simulink model "simscape_quadcopter_readtime_LQR_V1_2020a"  (R2022b)
settings: Solver=ode8  StartTime=0.0  StopTime=200  FixedStep=0.002  RelTol=1e-3
values from neighbouring files (symbols this model uses):
  C = [ 1  0  0  0  0  0 ... (first row only)    [LQR_QUADCOPTER_6STATE.m]    (also in LQR_QUADCOPTER_8STATE.m = [ 1     0     0     0     0     0     0     0)
  g = 9.81    [LQR_QUADCOPTER_6STATE.m]
  K_LQR_GOC = lqr(A,B,Q,R)    [LQR_QUADCOPTER_6STATE.m]
  m = 1.7    [LQR_QUADCOPTER_6STATE.m]
  pitch_init = 0    [LQR_QUADCOPTER_6STATE.m]    (also in LQR_QUADCOPTER_8STATE.m)
  roll_init = 0    [LQR_QUADCOPTER_6STATE.m]    (also in LQR_QUADCOPTER_8STATE.m)
  v_pitch_init = 0    [LQR_QUADCOPTER_6STATE.m]    (also in LQR_QUADCOPTER_8STATE.m)
  v_roll_init = 0    [LQR_QUADCOPTER_6STATE.m]    (also in LQR_QUADCOPTER_8STATE.m)
  v_x_init = 0    [LQR_QUADCOPTER_6STATE.m]    (also in LQR_QUADCOPTER_8STATE.m)
  v_y_init = 0    [LQR_QUADCOPTER_6STATE.m]    (also in LQR_QUADCOPTER_8STATE.m)
  v_yaw_init = 0    [LQR_QUADCOPTER_6STATE.m]    (also in LQR_QUADCOPTER_8STATE.m)
  v_z_init = 0    [LQR_QUADCOPTER_6STATE.m]    (also in LQR_QUADCOPTER_8STATE.m)
  x_init = 0    [LQR_QUADCOPTER_6STATE.m]    (also in LQR_QUADCOPTER_8STATE.m)
  y_init = 0    [LQR_QUADCOPTER_6STATE.m]    (also in LQR_QUADCOPTER_8STATE.m)
  yaw_init = 0    [LQR_QUADCOPTER_6STATE.m]    (also in LQR_QUADCOPTER_8STATE.m)
  z_init = 0    [LQR_QUADCOPTER_6STATE.m]    (also in LQR_QUADCOPTER_8STATE.m)
undefined symbols (not defined in the file or in its folder): drone_leg, X, Y, Z
libraries: sm_lib x55, nesl_utility x12, simulink x1
(part 2 of 2)

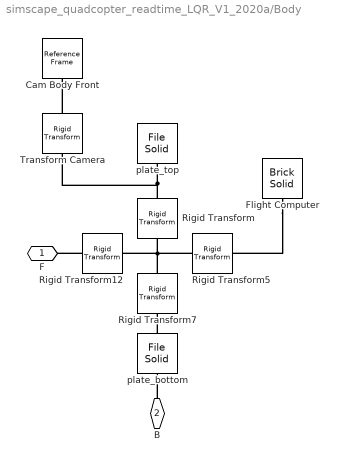
== system simscape_quadcopter_readtime_LQR_V1_2020a/Body ==
  Cam Body Front : sm_lib/Frames and Transforms/Reference Frame
  Flight Computer : sm_lib/Body Elements/Brick Solid  GraphicAmbientColor=[0.15 0.15 0.15 1.0]  BasedOnType=Mass  BrickDimensions=3*[20 20 5]  BrickDimensionUnits=mm  CenterOfMass=[0 0 0]  CenterOfMassUnits=m  GraphicDiffuseColor=[0.5 0.5 0.5]  Density=1000  DensityUnits=kg/m^3  DoExposeReferenceFrame=on  GraphicEmissiveColor=[0.0 0.0 0.0 1.0]  ExportEntireGeometry=off  SerializedFrames=<Frames/>  MarkerShape=Sphere  MarkerSize=10  GraphicType=FromGeometry  InertiaType=CalculateFromGeometry  Mass=638  MassUnits=g  MomentsOfInertia=[1 1 1]  MomentsOfInertiaUnits=kg*m^2  GraphicOpacity=1.0  ProductsOfInertia=[0 0 0]  ProductsOfInertiaUnits=kg*m^2  GraphicShininess=75  GraphicSpecularColor=[0.5 0.5 0.5 1.0]  GraphicVisPropType=SimpleVisualProperties
  Rigid Transform : sm_lib/Frames and Transforms/Rigid Transform  TranslationMethod=None  TranslationStandardOffset=0  TranslationLengthUnit=m  TranslationStandardAxis=+Z  TranslationCartesianOffset=[0 0 0]  TranslationROffset=0  TranslationROffsetUnits=m  TranslationZOffset=0  TranslationZOffsetUnits=m  TranslationThetaOffset=0  TranslationThetaOffsetUnits=deg  RotationMethod=None  RotationAngleUnits=deg  RotationStandardAxis=+Z  RotationAngle=45  RotationArbitraryAxis=[0 0 1]  FollAlignAxisA=+X  BaseAlignAxisA=+Y  FollAlignAxisB=+Y  BaseAlignAxisB=+Z  RotationSequenceAxes=FollowerAxes  RotationSequence=XYX  RotationSequenceAngles=[0 0 0]  RotationSequenceAnglesUnits=deg  RotationMatrix=[1 0 0; 0 1 0; 0 0 1]  Quaternion=[1 0 0 0]
  Rigid Transform12 : sm_lib/Frames and Transforms/Rigid Transform  TranslationMethod=Cartesian  TranslationStandardOffset=0  TranslationLengthUnit=mm  TranslationStandardAxis=+Z  TranslationCartesianOffset=[0 0 -26]  TranslationROffset=0  TranslationROffsetUnits=m  TranslationZOffset=0  TranslationZOffsetUnits=m  TranslationThetaOffset=0  TranslationThetaOffsetUnits=deg  RotationMethod=None  RotationAngleUnits=deg  RotationStandardAxis=+Z  RotationAngle=45  RotationArbitraryAxis=[0 0 1]  FollAlignAxisA=+X  BaseAlignAxisA=+Y  FollAlignAxisB=+Y  BaseAlignAxisB=+Z  RotationSequenceAxes=FollowerAxes  RotationSequence=XYX  RotationSequenceAngles=[0 0 0]  RotationSequenceAnglesUnits=deg  RotationMatrix=[1 0 0; 0 1 0; 0 0 1]  Quaternion=[1 0 0 0]
  Rigid Transform5 : sm_lib/Frames and Transforms/Rigid Transform  TranslationMethod=Cartesian  TranslationStandardOffset=0  TranslationLengthUnit=mm  TranslationStandardAxis=+Z  TranslationCartesianOffset=[0 0 -26]  TranslationROffset=0  TranslationROffsetUnits=m  TranslationZOffset=0  TranslationZOffsetUnits=m  TranslationThetaOffset=0  TranslationThetaOffsetUnits=deg  RotationMethod=None  RotationAngleUnits=deg  RotationStandardAxis=+Z  RotationAngle=45  RotationArbitraryAxis=[0 0 1]  FollAlignAxisA=+X  BaseAlignAxisA=+Y  FollAlignAxisB=+Y  BaseAlignAxisB=+Z  RotationSequenceAxes=FollowerAxes  RotationSequence=XYX  RotationSequenceAngles=[0 0 0]  RotationSequenceAnglesUnits=deg  RotationMatrix=[1 0 0; 0 1 0; 0 0 1]  Quaternion=[1 0 0 0]
  Rigid Transform7 : sm_lib/Frames and Transforms/Rigid Transform  TranslationMethod=Cartesian  TranslationStandardOffset=0  TranslationLengthUnit=mm  TranslationStandardAxis=+Z  TranslationCartesianOffset=[0 0 -38]  TranslationROffset=0  TranslationROffsetUnits=m  TranslationZOffset=0  TranslationZOffsetUnits=m  TranslationThetaOffset=0  TranslationThetaOffsetUnits=deg  RotationMethod=None  RotationAngleUnits=deg  RotationStandardAxis=+Z  RotationAngle=45  RotationArbitraryAxis=[0 0 1]  FollAlignAxisA=+X  BaseAlignAxisA=+Y  FollAlignAxisB=+Y  BaseAlignAxisB=+Z  RotationSequenceAxes=FollowerAxes  RotationSequence=XYX  RotationSequenceAngles=[0 0 0]  RotationSequenceAnglesUnits=deg  RotationMatrix=[1 0 0; 0 1 0; 0 0 1]  Quaternion=[1 0 0 0]
  Transform Camera : sm_lib/Frames and Transforms/Rigid Transform  TranslationMethod=Cartesian  TranslationStandardOffset=0  TranslationLengthUnit=m  TranslationStandardAxis=+Z  TranslationCartesianOffset=[0.06 0 0]  TranslationROffset=0  TranslationROffsetUnits=m  TranslationZOffset=0  TranslationZOffsetUnits=m  TranslationThetaOffset=0  TranslationThetaOffsetUnits=deg  RotationMethod=None  RotationAngleUnits=deg  RotationStandardAxis=+Z  RotationAngle=0.0  RotationArbitraryAxis=[0 0 1]  FollAlignAxisA=+X  BaseAlignAxisA=+Y  FollAlignAxisB=+Y  BaseAlignAxisB=+Z  RotationSequenceAxes=FollowerAxes  RotationSequence=XYX  RotationSequenceAngles=[0 0 0]  RotationSequenceAnglesUnits=deg  RotationMatrix=[1 0 0; 0 1 0; 0 0 1]  Quaternion=[1 0 0 0]
  plate_bottom : sm_lib/Body Elements/File Solid  ExtGeomFileName=C:\Users\tridu\OneDrive\Máy tính\(1)\mohinh\quadcopter_simscape\Quadcopter-Simulation-master\Quadcopter-Simulation-master\CAD\Geometry\quadcopter_drone_plate_bottom.stp  UnitType=FromFile  ExtGeomFileUnits=m  StepReaderType=HEX  ExportConvexHullGeometry=off  InertiaType=Custom  Mass=0.0317292  MassUnits=kg  CenterOfMass=[9.57262e-08, 1.0716e-07, -1.47882e-10]  CenterOfMassUnits=m  MomentsOfInertia=[2.77785e-05, 2.75764e-05, 5.53432e-05]  MomentsOfInertiaUnits=kg*m^2  ProductsOfInertia=[-9.24719e-13, -9.71809e-13, 1.0181e-10]  ProductsOfInertiaUnits=kg*m^2  BasedOnType=Density  Density=1  DensityUnits=g/cm^3  DoExposeReferenceFrame=off  SerializedFrames=<Frames><Frame><Id>Frame1</Id><Value><Name>Bot</Name><Origin><Source>GeometricFeature</Source><FeatureName>planar surface 33</FeatureName></Origin><PrimaryAxis><DefinedDirection>+Z</DefinedDirection><Source>ReferenceFrame</Source><SourceDirection>+Z</SourceDirection><FeatureName></FeatureName></PrimaryAxis><SecondaryAxis><DefinedDirection>+X</DefinedDirection><Source>ReferenceFrame</Source><SourceDirection>+Y</SourceDirection><FeatureName></FeatureName></SecondaryAxis></Value></Frame><Frame><Id>Frame2</Id><Value><Name>Top</Name><Origin><Source>ReferenceFrame</Source><FeatureName></FeatureName></Origin><PrimaryAxis><DefinedDirection>+Z</DefinedDirection><Source>ReferenceFrame</Source><SourceDirection>+Z</SourceDirection><FeatureName></FeatureName></PrimaryAxis><SecondaryAxis><DefinedDirection>+X</DefinedDirection><Source>ReferenceFrame</Source><SourceDirection>+Y</SourceDirection><FeatureName></FeatureName></SecondaryAxis></Value></Frame></Frames>  GraphicType=FromGeometry  MarkerShape=Sphere  MarkerSize=10  GraphicVisPropType=SimpleVisualProperties  GraphicDiffuseColor=[0.0 0.0 0.0]  GraphicSpecularColor=[0.5 0.5 0.5 1.0]  GraphicAmbientColor=[0.15 0.15 0.15 1.0]  GraphicEmissiveColor=[0.0 0.0 0.0 1.0]  GraphicShininess=75  GraphicOpacity=1.0
  "plate_top " : sm_lib/Body Elements/File Solid  ExtGeomFileName=C:\Users\tridu\OneDrive\Máy tính\(1)\mohinh\quadcopter_simscape\Quadcopter-Simulation-master\Quadcopter-Simulation-master\CAD\Geometry\quadcopter_drone_plate_top.stp  UnitType=FromFile  ExtGeomFileUnits=m  StepReaderType=HEX  ExportConvexHullGeometry=off  InertiaType=Custom  Mass=0.0317292  MassUnits=kg  CenterOfMass=[9.57262e-08, 1.0716e-07, -1.47882e-10]  CenterOfMassUnits=m  MomentsOfInertia=[2.77785e-05, 2.75764e-05, 5.53432e-05]  MomentsOfInertiaUnits=kg*m^2  ProductsOfInertia=[-9.24719e-13, -9.71809e-13, 1.0181e-10]  ProductsOfInertiaUnits=kg*m^2  BasedOnType=Density  Density=1  DensityUnits=g/cm^3  DoExposeReferenceFrame=on  SerializedFrames=<Frames/>  GraphicType=FromGeometry  MarkerShape=Sphere  MarkerSize=10  GraphicVisPropType=SimpleVisualProperties  GraphicDiffuseColor=[0.0 0.0 0.0]  GraphicSpecularColor=[0.5 0.5 0.5 1.0]  GraphicAmbientColor=[0.15 0.15 0.15 1.0]  GraphicEmissiveColor=[0.0 0.0 0.0 1.0]  GraphicShininess=75  GraphicOpacity=1.0
  F : PMIOPort  Side=Right
  B : PMIOPort  Port=2  Side=Left
  connections:
  Flight Computer/RConn1 -- Rigid Transform5/RConn1
  Rigid Transform7/LConn1 -- Rigid Transform5/LConn1 -- Rigid Transform12/LConn1 -- Rigid Transform/LConn1
  plate_bottom/RConn1 -- Rigid Transform7/RConn1
  Rigid Transform12/RConn1 -- F/RConn1
  Rigid Transform/RConn1 -- Transform Camera/LConn1 -- "plate_top "/RConn1
  Transform Camera/RConn1 -- Cam Body Front/RConn1
  B/RConn1 -- plate_bottom/LConn1

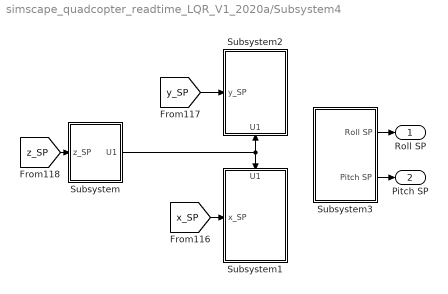
== system simscape_quadcopter_readtime_LQR_V1_2020a/Subsystem4 ==
  Subsystem : Subsystem
  Subsystem1 : Subsystem
      settings: PortSchema="{\"entries\":[{\"content\":{\"sides\":[{\"content\":{\"connectorIds\":[\"In1\"]},\"type\":\"ConnectorPlacement.EquallySpacedRectSide\",\"uuid\":\"62a51b67-9663-4f23-a0a7-17dd4d665e7c\"},{\"content\":{\"connectorIds\":[],\"side\":\"RIGHT\"},\"type\":\"ConnectorPlacement.EquallySpacedRectSide\",\"uuid\":\"9cf76029-abe2-4d70-b924-e49b8fca58fe\"},{\"content\":{\"connectorIds\":[\"In2\"],\"side\":\"TOP\"},\"type\":\"ConnectorPlacement.EquallySpacedRectSide\",\"uuid\":\"b4a1b99f-921e-474f-a2a2-454a2b8db441\"}]},\"type\":\"ConnectorPlacement.EquallySpacedConnector\",\"uuid\":\"20d905bc-00f9-441a-91aa-89485326b1f1\"}],\"packageUris\":[\"http://schema.mathworks.com/mf0/Connector/R2020b\"],\"version\":\"1.0\"}"
  Subsystem2 : Subsystem
      settings: PortSchema="{\"entries\":[{\"content\":{\"sides\":[{\"content\":{\"connectorIds\":[\"In1\"]},\"type\":\"ConnectorPlacement.EquallySpacedRectSide\",\"uuid\":\"62a51b67-9663-4f23-a0a7-17dd4d665e7c\"},{\"content\":{\"connectorIds\":[],\"side\":\"RIGHT\"},\"type\":\"ConnectorPlacement.EquallySpacedRectSide\",\"uuid\":\"9cf76029-abe2-4d70-b924-e49b8fca58fe\"},{\"content\":{\"connectorIds\":[],\"side\":\"TOP\"},\"type\":\"ConnectorPlacement.EquallySpacedRectSide\",\"uuid\":\"b4a1b99f-921e-474f-a2a2-454a2b8db441\"},{\"content\":{\"connectorIds\":[\"In2\"],\"side\":\"BOTTOM\"},\"type\":\"ConnectorPlacement.EquallySpacedRectSide\",\"uuid\":\"85e13e03-6c73-4551-a07f-9b1bfbaf7196\"}]},\"type\":\"ConnectorPlacement.EquallySpacedConnector\",\"uuid\":\"20d905bc-00f9-441a-91aa-89485326b1f1\"}],\"packageUris\":[\"http://schema.mathworks.com/mf0/Connector/R2020b\"],\"version\":\"1.0\"}"
  Subsystem3 : Subsystem
  Roll SP : Outport
  Pitch SP : Outport  Port=2
  wires:
  Subsystem3/2(Pitch SP) -> Pitch SP/1
  [z_SP] -> Subsystem/1(z_SP)
  [y_SP] -> Subsystem2/1(y_SP)
  Subsystem3/1(Roll SP) -> Roll SP/1
  [x_SP] -> Subsystem1/1(x_SP)
  Subsystem/1(U1) -> Subsystem1/2(U1), Subsystem2/2(U1)

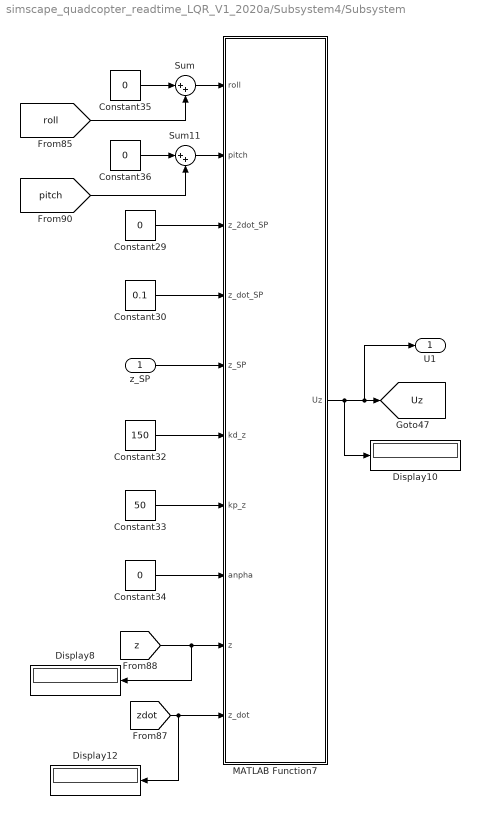
== system simscape_quadcopter_readtime_LQR_V1_2020a/Subsystem4/Subsystem ==
  z_SP : Inport
  Constant{29,34..36} (4 alike) : Constant  Value=0
  Constant30 : Constant  Value=0.1
  Constant32 : Constant  Value=150
  Constant33 : Constant  Value=50
  Display10 : Display
  Display12 : Display
  Display8 : Display
  MATLAB Function7 : MATLAB Function  TreatAsAtomicUnit=on
  Sum : Sum  Inputs=|++
  Sum11 : Sum  Inputs=|++
  U1 : Outport
  tag scope: Uz=global
  wires:
  [z] -> Display8/1, MATLAB Function7/9(z)
  Constant35/1 -> Sum/1
  Constant29/1 -> MATLAB Function7/3(z_2dot_SP)
  Constant32/1 -> MATLAB Function7/6(kd_z)
  Constant30/1 -> MATLAB Function7/4(z_dot_SP)
  [zdot] -> Display12/1, MATLAB Function7/10(z_dot)
  Sum11/1 -> MATLAB Function7/2(pitch)
  [roll] -> Sum/2
  Constant34/1 -> MATLAB Function7/8(anpha)
  Constant33/1 -> MATLAB Function7/7(kp_z)
  [pitch] -> Sum11/2
  Sum/1 -> MATLAB Function7/1(roll)
  MATLAB Function7/1(Uz) -> Display10/1, U1/1, [Uz]
  Constant36/1 -> Sum11/1
  z_SP/1 -> MATLAB Function7/5(z_SP)

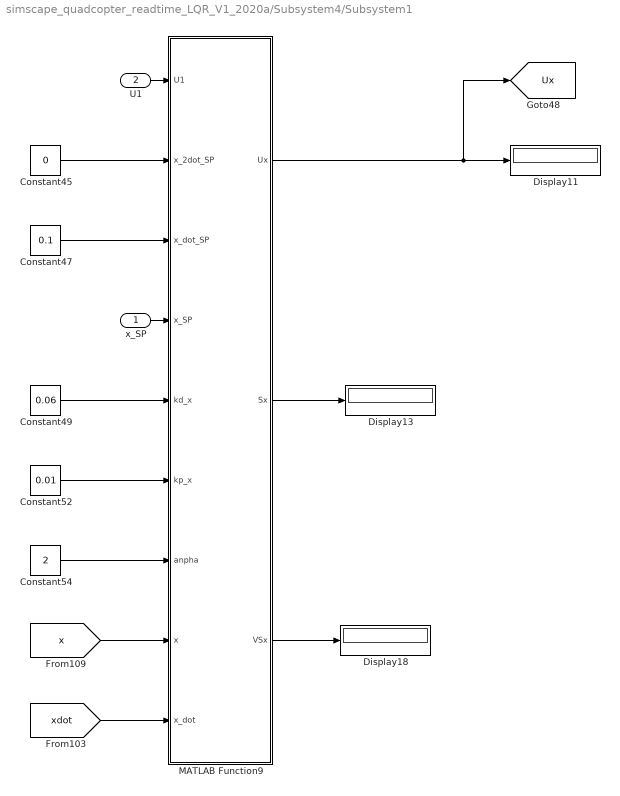
== system simscape_quadcopter_readtime_LQR_V1_2020a/Subsystem4/Subsystem1 ==
  x_SP : Inport
  U1 : Inport  Port=2
  Constant45 : Constant  Value=0
  Constant47 : Constant  Value=0.1
  Constant49 : Constant  Value=0.06
  Constant52 : Constant  Value=0.01
  Constant54 : Constant  Value=2
  Display11 : Display
  Display13 : Display
  Display18 : Display
  MATLAB Function9 : MATLAB Function  TreatAsAtomicUnit=on
  tag scope: Ux=global
  wires:
  Constant49/1 -> MATLAB Function9/5(kd_x)
  Constant54/1 -> MATLAB Function9/7(anpha)
  U1/1 -> MATLAB Function9/1(U1)
  MATLAB Function9/3(VSx) -> Display18/1
  MATLAB Function9/2(Sx) -> Display13/1
  [x] -> MATLAB Function9/8(x)
  Constant52/1 -> MATLAB Function9/6(kp_x)
  [xdot] -> MATLAB Function9/9(x_dot)
  Constant45/1 -> MATLAB Function9/2(x_2dot_SP)
  Constant47/1 -> MATLAB Function9/3(x_dot_SP)
  x_SP/1 -> MATLAB Function9/4(x_SP)
  MATLAB Function9/1(Ux) -> Display11/1, [Ux]

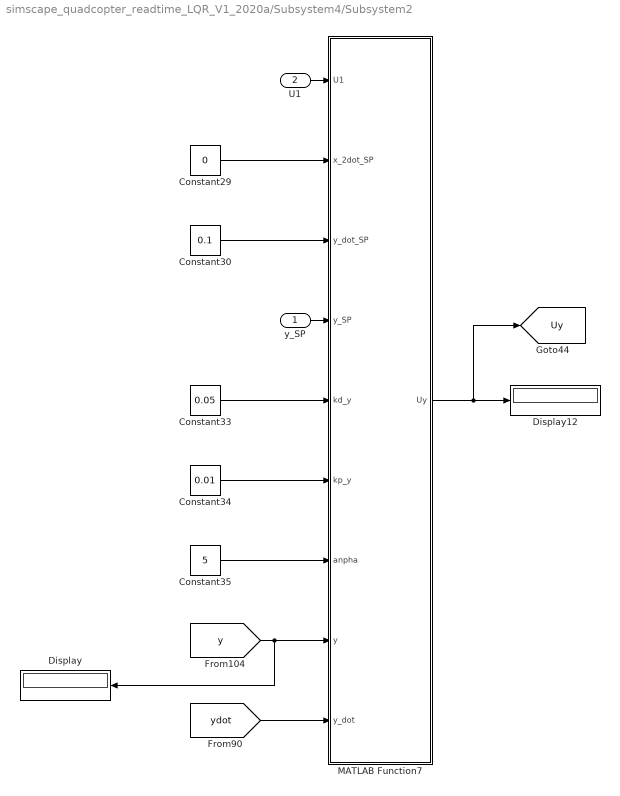
== system simscape_quadcopter_readtime_LQR_V1_2020a/Subsystem4/Subsystem2 ==
  y_SP : Inport
  U1 : Inport  Port=2
  Constant29 : Constant  Value=0
  Constant30 : Constant  Value=0.1
  Constant33 : Constant  Value=0.05
  Constant34 : Constant  Value=0.01
  Constant35 : Constant  Value=5
  Display : Display
  Display12 : Display
  MATLAB Function7 : MATLAB Function  TreatAsAtomicUnit=on
  tag scope: Uy=global
  wires:
  [ydot] -> MATLAB Function7/9(y_dot)
  Constant35/1 -> MATLAB Function7/7(anpha)
  Constant29/1 -> MATLAB Function7/2(x_2dot_SP)
  Constant34/1 -> MATLAB Function7/6(kp_y)
  MATLAB Function7/1(Uy) -> Display12/1, [Uy]
  Constant33/1 -> MATLAB Function7/5(kd_y)
  U1/1 -> MATLAB Function7/1(U1)
  Constant30/1 -> MATLAB Function7/3(y_dot_SP)
  y_SP/1 -> MATLAB Function7/4(y_SP)
  [y] -> Display/1, MATLAB Function7/8(y)

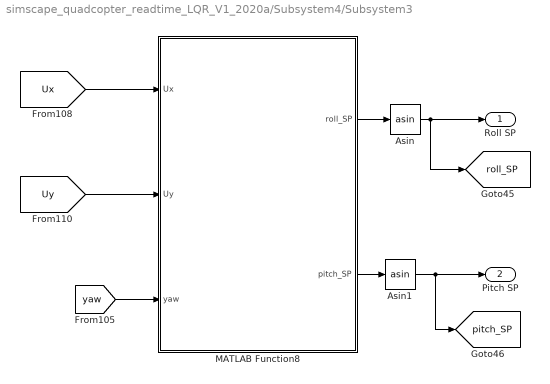
== system simscape_quadcopter_readtime_LQR_V1_2020a/Subsystem4/Subsystem3 ==
  Asin : Trigonometry  Operator=asin
  Asin1 : Trigonometry  Operator=asin
  MATLAB Function8 : MATLAB Function  TreatAsAtomicUnit=on
  Roll SP : Outport
  Pitch SP : Outport  Port=2
  tag scope: pitch_SP=global, roll_SP=global
  wires:
  [Ux] -> MATLAB Function8/1(Ux)
  [Uy] -> MATLAB Function8/2(Uy)
  MATLAB Function8/1(roll_SP) -> Asin/1
  Asin/1 -> Roll SP/1, [roll_SP]
  Asin1/1 -> [pitch_SP], Pitch SP/1
  [yaw] -> MATLAB Function8/3(yaw)
  MATLAB Function8/2(pitch_SP) -> Asin1/1

== matlab function simscape_quadcopter_readtime_LQR_V1_2020a/Subsystem4/Subsystem2/MATLAB Function7 ==
  data: U1 input; x_2dot_SP input; y_dot_SP input; y_SP input; kd_y input; kp_y input; Uy output; anpha input; y input; y_dot input
function Uy = fcn(U1,x_2dot_SP,y_dot_SP,y_SP,kd_y,kp_y,anpha,y,y_dot) 

%% khai báo biến hệ thống
m=1.7;

%% phương trình trạng thái

% y_2dot=-(U1*cos(yaw)*sin(roll) - cos(roll)*sin(pitch)*sin(yaw))/m;

%% Chọn phương trình mặt trượt có dạng

Sy=kd_y*(y_dot_SP-y_dot)+kp_y*(y_SP-y);

%% Chọn tiêu chí tốc độ hội tụ, trong đó K là hệ số dương Nếu K càng lớn thì độ hội tụ về 0 càng giảm

VSy=-anpha*abs(Sy)*sign(Sy);

%% Thiết kế tín hiệu điều khiển Ux Uy

Uy=(m/U1)*(x_2dot_SP+Sy+VSy);

end

== matlab function simscape_quadcopter_readtime_LQR_V1_2020a/Subsystem4/Subsystem1/MATLAB Function9 ==
  data: U1 input; x_2dot_SP input; x_dot_SP input; x_SP input; kd_x input; kp_x input; Ux output; anpha input; x input; x_dot input; Sx output; VSx output
function [Ux,Sx,VSx]= fcn(U1,x_2dot_SP,x_dot_SP,x_SP,kd_x,kp_x,anpha,x,x_dot) 

%% khai báo biến hệ thống

m=1.7;

%% phương trình trạng thái

% x_2dot=(U1*sin(roll)*sin(yaw) + cos(roll)*cos(yaw)*sin(pitch))/m;

%% Chọn phương trình mặt trượt có dạng

Sx=kd_x*(x_dot_SP-x_dot)+kp_x*(x_SP-x);

%% Chọn tiêu chí tốc độ hội tụ, trong đó K là hệ số dương Nếu K càng lớn thì độ hội tụ về 0 càng giảm

VSx=-anpha*abs(Sx)*sign(Sx);

%% Thiết kế tín hiệu điều khiển Ux Uy

Ux=(m/U1)*(x_2dot_SP+Sx+VSx);

end

== matlab function simscape_quadcopter_readtime_LQR_V1_2020a/Subsystem4/Subsystem3/MATLAB Function8 ==
  data: Ux input; roll_SP output; Uy input; yaw input; pitch_SP output
function [roll_SP,pitch_SP]= fcn(Ux,Uy,yaw)

roll_SP_tt=(Uy*cos(yaw))/(cos(yaw)^2 + sin(yaw)^2) + (Ux*sin(yaw))/(cos(yaw)^2 + sin(yaw)^2);

pitch_SP=((Uy*sin(yaw))/(cos(yaw)^2 + sin(yaw)^2) - (Ux*cos(yaw))/(cos(yaw)^2 + sin(yaw)^2))/cos(roll_SP_tt);

roll_SP=roll_SP_tt;

end

== matlab function simscape_quadcopter_readtime_LQR_V1_2020a/MATLAB Function1 ==
  data: D1 input; T1 output; D2 input; D3 input; D4 input; T2 output; T3 output; T4 output
function [T1,T2,T3,T4]= fcn(D1,D2,D3,D4)
T1=(D1-1000)/1000*11.5;
T2=(D2-1000)/1000*11.5;
T3=(D3-1000)/1000*11.5;
T4=(D4-1000)/1000*11.5;

end

== matlab function simscape_quadcopter_readtime_LQR_V1_2020a/MATLAB Function ==
  data: T1 input; x2dot output; T2 input; T3 input; T4 input; roll input; pitch input; yaw input; roll_dot input; pitch_dot input; yaw_dot input; y2dot output; z2dot output; roll2dot output; pitch2dot output; yaw2dot output; HS_MSKK input; x_dot input; y_dot input; z_dot input
function [x2dot,y2dot,z2dot,roll2dot,pitch2dot,yaw2dot]= fcn(T1,T2,T3,T4,roll,pitch,yaw,roll_dot,pitch_dot,yaw_dot,HS_MSKK,x_dot,y_dot,z_dot)
    m = 1.7; %kg
    l = 0.25; %m
    % % b = 4.74E-5;
    % % d = 2.35E-7;
    g = 9.81; %ms2
    % % to = 0.05; %Nm
    Ix = 0.0030842; %kg.m2
    Iy = 0.0030842; %kg.m2
    Iz = 0.0032315; %kg.m2
    % Ir = 1E-4; %kg.m2
    U1 = T1+T2+T3+T4;
    U2 = l*(T2-T4);
    U3 = l*(T3-T1);
    U4 = T1-T2+T3-T4;

    x2dot=(U1*(sin(roll)*sin(yaw) + cos(roll)*cos(yaw)*sin(pitch)))/m;
    y2dot=-(U1*(cos(yaw)*sin(roll) - cos(roll)*sin(pitch)*sin(yaw)))/m;
    z2dot=(U1*cos(pitch)*cos(roll))/m - g;
    roll2dot=(Iy*pitch_dot*yaw_dot - Iz*pitch_dot*yaw_dot)/Ix + U2/Ix;
    pitch2dot=U3/Iy + (-Ix*roll_dot*yaw_dot + Iz*roll_dot*yaw_dot)/Iy;
    yaw2dot=U4/Iz + (Ix*pitch_dot*roll_dot - Iy*pitch_dot*roll_dot)/Iz;

% %% Gia lap ma sat theo cong thuc ma sat tuyen tinh voi he so cho truoc la
    FX_Friction     =  -  HS_MSKK * x_dot;
    FY_Friction     =  -  HS_MSKK * y_dot;
    FZ_Friction     =  -  HS_MSKK * z_dot;
    FR_Friction     =  -  HS_MSKK * roll_dot;
    FP_Friction     =  -  HS_MSKK * pitch_dot;
    FYaw_Friction   =  -  HS_MSKK * yaw_dot;
    FX_Limit        =     HS_MSKK /10;
    FY_Limit        =     HS_MSKK /10;
    FZ_Limit        =     HS_MSKK /10;
    FR_Limit        =     HS_MSKK /10;
    FP_Limit        =     HS_MSKK /10;
    FYaw_Limit      =     HS_MSKK /10;
    
    if(FX_Friction > FX_Limit)
        FX_Friction = FX_Limit;
    end
    if(FX_Friction < -FX_Limit)
        FX_Friction = -FX_Limit;
    end
    
    if(FY_Friction > FY_Limit)
        FY_Friction = FY_Limit;
    end
    if(FY_Friction < -FY_Limit)
        FY_Friction = -FY_Limit;
    end
    
    if(FZ_Friction > FZ_Limit)
        FZ_Friction = FZ_Limit;
    end
    if(FZ_Friction < -FZ_Limit)
        FZ_Friction = -FZ_Limit;
    end
    
    if(FR_Friction > FR_Limit)
        FR_Friction = FR_Limit;
    end
    if(FR_Friction < -FR_Limit)
        FR_Friction = -FR_Limit;
    end
    
    if(FP_Friction > FP_Limit)
        FP_Friction = FP_Limit;
    end
    if(FP_Friction < -FP_Limit)
        FP_Friction = -FP_Limit;
    end
    
    if(FYaw_Friction > FYaw_Limit)
        FYaw_Friction = FYaw_Limit;
    end
    if(FYaw_Friction < -FYaw_Limit)
        FYaw_Friction = -FYaw_Limit;
    end
    
    F_x2dot           = m*x2dot     - FX_Friction;
    if((m*x2dot)*(F_x2dot)<=0)
        F_x2dot     = m*x2dot;
    end
    F_y2dot           = m*y2dot     - FY_Friction;
    if((m*y2dot)*(F_y2dot)<=0)
        F_y2dot     = m*y2dot;
    end
    F_z2dot           = m*z2dot     - FZ_Friction;
    if((m*z2dot)*(F_z2dot)<=0)
        F_z2dot     = m*z2dot;
    end
    F_roll2dot        = m*roll2dot  - FR_Friction;
    if((m*roll2dot)*(F_roll2dot)<=0)
        F_roll2dot  = m*roll2dot;
    end
    F_pitch2dot       = m*pitch2dot - FP_Friction;
    if((m*pitch2dot)*(F_pitch2dot)<=0)
        F_pitch2dot = m*pitch2dot;
    end
    F_yaw2dot         = m*yaw2dot   - FYaw_Friction;
    if((m*yaw2dot)*(F_yaw2dot)<=0)
        F_yaw2dot   = m*yaw2dot;
    end

    x2dot           = F_x2dot/m;
    y2dot           = F_y2dot/m;
    z2dot           = F_z2dot/m;
    roll2dot        = F_roll2dot/m;
    pitch2dot       = F_pitch2dot/m;
    yaw2dot         = F_yaw2dot/m;
end

== matlab function simscape_quadcopter_readtime_LQR_V1_2020a/MATLAB Function2 ==
  data: T1 input; D1 output; T2 input; T3 input; T4 input; D2 output; D3 output; D4 output
function [D1,D2,D3,D4]= fcn(T1,T2,T3,T4)
D1=(T1/11.5)*1000+1000;
D2=(T2/11.5)*1000+1000;
D3=(T3/11.5)*1000+1000;
D4=(T4/11.5)*1000+1000;

end

== matlab function simscape_quadcopter_readtime_LQR_V1_2020a/Subsystem4/Subsystem/MATLAB Function7 ==
  settings: updateMethod=DISCRETE
  data: roll input; pitch input; z_2dot_SP input; z_dot_SP input; z_SP input; kd_z input; kp_z input; anpha input; z input; z_dot input; Uz output
function Uz = fcn(roll,pitch,z_2dot_SP,z_dot_SP,z_SP,kd_z,kp_z,anpha,z,z_dot) 
persistent U1 
%% khai báo biến hệ thống
g=9.81;
m=1.7;

if isempty(U1)    
    U1 = 0;
end

%% phương trình trạng thái

z_2dot=(U1*cos(pitch)*cos(roll))/m - g;

%% Chọn phương trình mặt trượt có dạng

Sz=(z_2dot_SP-z_2dot)+kd_z*(z_dot_SP-z_dot)+kp_z*(z_SP-z);

%% Chọn tiêu chí tốc độ hội tụ, trong đó K là hệ số dương Nếu K càng lớn thì độ hội tụ về 0 càng giảm

VSz_dot=-anpha*abs(kd_z*(z_dot_SP-z_dot)+kp_z*(z_SP-z))*sign(kd_z*(z_dot_SP-z_dot)+kp_z*(z_SP-z));

%% Thiết kế tín hiệu điều khiển Ux Uy

Uz=(m/(cos(roll)*cos(pitch)))*(g+z_2dot_SP+kd_z*(z_dot_SP-z_dot)+kp_z*(z_SP-z)+VSz_dot);


if (Uz==m*g)
    Uz=0;
end
end
